simulink model "configB"  (R2022b)
settings: Solver=VariableStepAuto  StartTime=0.0  StopTime=150  RelTol=1e-3
values from neighbouring files (symbols this model uses):
  densityHydrogen = poutlet*(molarMassHydrogen/1000)/(universalGasConstant2*0.001)/OperatingTemperature    (= 0.0969930238153)    [ValveSetData.m]
  flowCoefficientValve = 1.156 * 0.32    (= 0.36992)    [ValveSetData.m]
  hysteresisValve = 0.15    [ValveSetData.m]
  molarMassHydrogen = 2.016    [ValveSetData.m]
  N2 = 6950    [ValveSetData.m]
  OperatingTemperature = T_S+27    (= 300)    [ValveSetData.m]
  responseTimeValve = 0.03    [ValveSetData.m]
  SpecificGravityHydrogen = 0.0696    [ValveSetData.m]
  universalGasConstant1 = 8.3145    [ValveSetData.m]
undefined symbols (not defined in the file or in its folder): anodeInletPathVolume
libraries: slpidlib x1
settings Model: Creator=debjani.ghosh  LastModifiedBy=debjani.ghosh
settings DataIOCC: ReturnWorkspaceOutputs=off

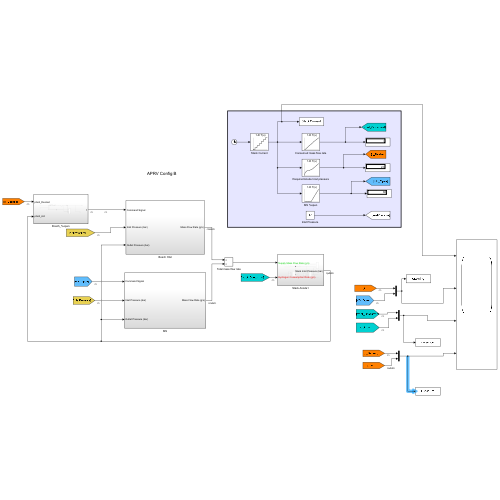
[thumbnail: Simulink's stored preview of the top-level diagram]
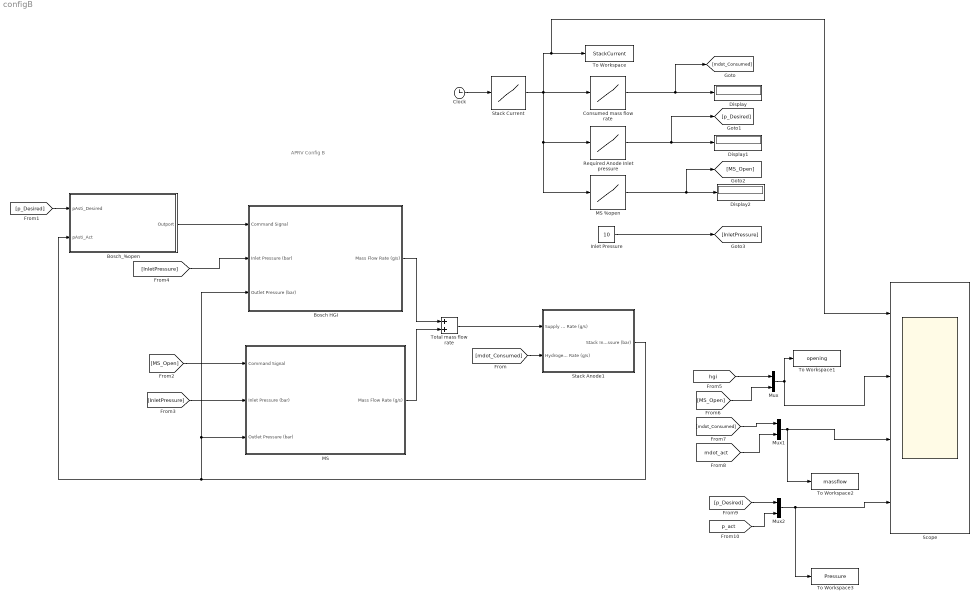
== system configB ==
  note: APRV Config B
  Bosch HGI : Subsystem
  Bosch_%open : Subsystem
  Clock : Clock
  Consumed mass flow rate : Lookup_n-D  NumberOfTableDimensions=1  BreakpointsForDimension1=[0;20;100;200;300;400;500;600]  Table=[0;0.1;0.5;1;1.5;2;2.5;3]  InternalRulePriority=Speed  RndMeth=Simplest
  Display : Display
  Display1 : Display
  Display2 : Display
  Inlet Pressure : Constant  Value=10
  MS : Subsystem
  MS %open : Lookup_n-D  NumberOfTableDimensions=1  BreakpointsForDimension1=[20,100,200,300,400,500,600]  Table=[0;0;0;0;20;40;60]  InternalRulePriority=Speed  RndMeth=Simplest
  Mux : Mux  Inputs=2
  Mux1 : Mux  Inputs=2
  Mux2 : Mux  Inputs=2
  Required Anode Inlet pressure : Lookup_n-D  NumberOfTableDimensions=1  BreakpointsForDimension1=[0;20;100;200;300;400;500;600]  Table=[1;1.4;1.6;1.7;1.8;2;2.3;2.6]  InternalRulePriority=Speed  RndMeth=Simplest
  Scope : Scope  NumInputPorts=4
  Stack Anode1 : Subsystem
  Stack Current : Lookup_n-D  NumberOfTableDimensions=1  BreakpointsForDimension1=[0;3;5.8;20;21.6;42;44;64;66;86;88;108;110;130;132;150]  Table=[0;0;20;20;100;100;200;200;300;300;400;400;500;500;600;600]  InternalRulePriority=Speed  RndMeth=Simplest
  To Workspace : ToWorkspace  VariableName=StackCurrent  SaveFormat=Structure With Time  SampleTime=-1
  To Workspace1 : ToWorkspace  VariableName=opening  SaveFormat=Structure With Time  SampleTime=-1
  To Workspace2 : ToWorkspace  VariableName=massflow  SaveFormat=Structure With Time  SampleTime=-1
  To Workspace3 : ToWorkspace  VariableName=Pressure  SaveFormat=Structure With Time  SampleTime=-1
  Total mass flow rate : Sum
  wires:
  [InletPressure] -> MS/2(Inlet Pressure (bar))
  Stack Anode1/1(Stack Inlet Pressure (bar)) -> Bosch_%open/2(pAsti_Act), Bosch HGI/3(Outlet Pressure (bar)), MS/3(Outlet Pressure (bar))
  MS/1(Mass Flow Rate (g/s)) -> Total mass flow rate/2
  Bosch_%open/1(Outport) -> Bosch HGI/1("Command Signal ")
  Bosch HGI/1(Mass Flow Rate (g/s)) -> Total mass flow rate/1
  Total mass flow rate/1 -> Stack Anode1/1(Supply Mass Flow Rate (g/s))
  Consumed mass flow rate/1 -> [mdot_Consumed], Display/1
  Required Anode Inlet pressure/1 -> [p_Desired], Display1/1
  [p_Desired] -> Bosch_%open/1(pAsti_Desired)
  [MS_Open] -> MS/1("Command Signal ")
  [mdot_Consumed] -> Stack Anode1/2(Hydrogen Consumption Rate (g/s))
  Clock/1 -> Stack Current/1
  MS %open/1 -> [MS_Open], Display2/1
  Stack Current/1 -> MS %open/1, Required Anode Inlet pressure/1, Scope/1, To Workspace/1, Consumed mass flow rate/1
  [InletPressure] -> Bosch HGI/2(Inlet Pressure (bar))
  Inlet Pressure/1 -> [InletPressure]
  Mux/1 -> To Workspace1/1, Scope/2
  [hgi] -> Mux/1
  [MS_Open] -> Mux/2
  [mdot_Consumed] -> Mux1/1
  [mdot_act] -> Mux1/2
  [p_Desired] -> Mux2/1
  Mux1/1 -> To Workspace2/1, Scope/3
  [p_act] -> Mux2/2
  Mux2/1 -> To Workspace3/1, Scope/4

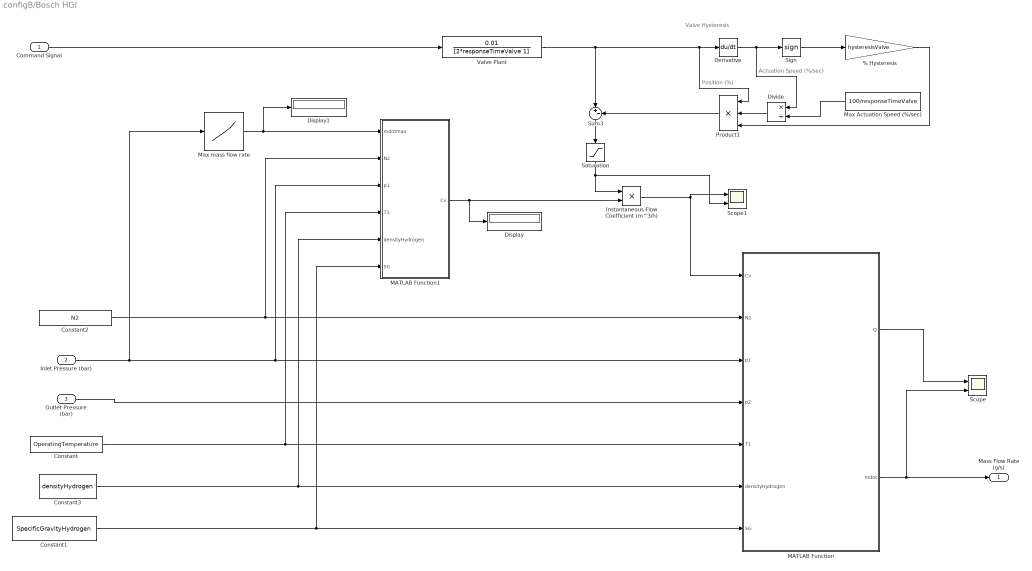
== system configB/Bosch HGI ==
  note: Actuation Speed (%/sec)
  note: Position (%)
  note: Valve Hysteresis
  "Command Signal " : Inport
  Inlet Pressure (bar) : Inport  Port=2
  Outlet Pressure (bar) : Inport  Port=3
  % Hysteresis : Gain  Gain=hysteresisValve
  Constant : Constant  Value=OperatingTemperature
  Constant1 : Constant  Value=SpecificGravityHydrogen
  Constant2 : Constant  Value=N2
  Constant3 : Constant  Value=densityHydrogen
  Derivative : Derivative
  Display : Display
  Display1 : Display
  Divide : Product  Inputs=*/
  Instantaneous Flow Coefficient (m^3/h) : Product
  MATLAB Function : MATLAB Function  TreatAsAtomicUnit=on
  MATLAB Function1 : MATLAB Function  TreatAsAtomicUnit=on
  Max Actuation Speed (%/sec) : Constant  Value=100/responseTimeValve
  Max mass flow rate : Lookup_n-D  NumberOfTableDimensions=1  BreakpointsForDimension1=[8,10,12,14,16]  Table=[1.5,1.8,2.2,2.5,2.8]  InternalRulePriority=Speed  RndMeth=Simplest
  Product1 : Product  Inputs=3
  Saturation : Saturate  UpperLimit=1  LowerLimit=0  LinearizeAsGain=off
  Scope : Scope  NumInputPorts=2
  Scope1 : Scope  NumInputPorts=2
  Sign : Signum  ZeroCross=off
  Sum3 : Sum  Inputs=|+-
  Valve Plant : TransferFcn  Numerator=0.01  Denominator=[2*responseTimeValve 1]
  Mass Flow Rate (g/s) : Outport
  wires:
  Sign/1 -> % Hysteresis/1
  Derivative/1 -> Divide/1, Sign/1
  % Hysteresis/1 -> Product1/3
  Product1/1 -> Sum3/2
  Sum3/1 -> Saturation/1
  Divide/1 -> Product1/2
  Max Actuation Speed (%/sec)/1 -> Divide/2
  Instantaneous Flow Coefficient (m^3/h)/1 -> MATLAB Function/1(Cv), Scope1/1
  Valve Plant/1 -> Sum3/1, Derivative/1, Product1/1
  "Command Signal "/1 -> Valve Plant/1
  MATLAB Function/2(mdot) -> Scope/2, Mass Flow Rate (g/s)/1
  Saturation/1 -> Scope1/2, Instantaneous Flow Coefficient (m^3/h)/1
  Constant1/1 -> MATLAB Function1/6(SG), MATLAB Function/7(SG)
  Constant/1 -> MATLAB Function/5(T1), MATLAB Function1/4(T1)
  Outlet Pressure (bar)/1 -> MATLAB Function/4(p2)
  MATLAB Function1/1(Cv) -> Display/1, Instantaneous Flow Coefficient (m^3/h)/2
  Constant2/1 -> MATLAB Function1/2(N2), MATLAB Function/2(N2)
  Inlet Pressure (bar)/1 -> Max mass flow rate/1, MATLAB Function1/3(p1), MATLAB Function/3(p1)
  Max mass flow rate/1 -> Display1/1, MATLAB Function1/1(mdotmax)
  Constant3/1 -> MATLAB Function1/5(densityHydrogen), MATLAB Function/6(densityHydrogen)
  MATLAB Function/1(Q) -> Scope/1

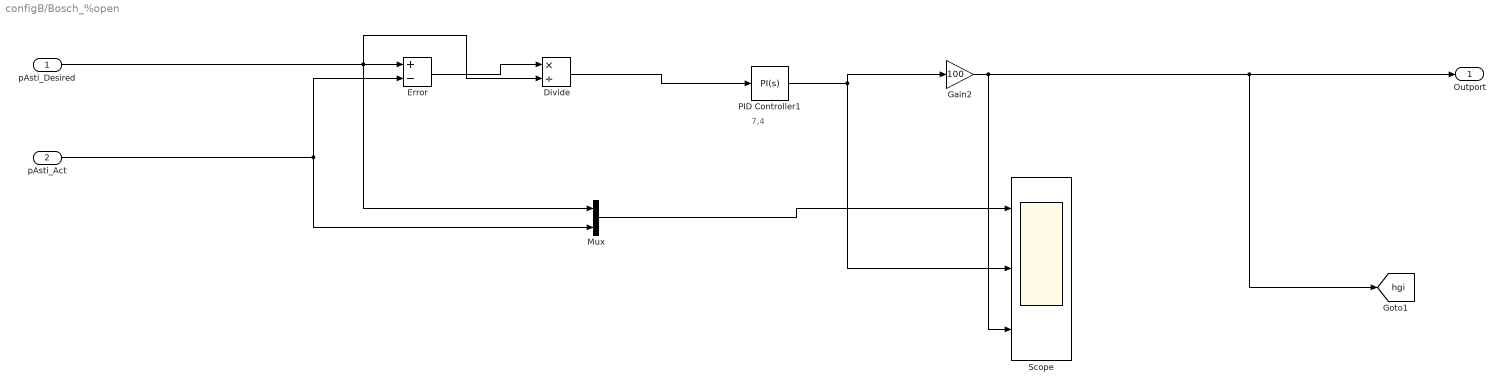
== system configB/Bosch_%open ==
  note: 7,4
  pAsti_Desired : Inport
  pAsti_Act : Inport  Port=2
  Divide : Product  Inputs=*/
  Error : Sum  Inputs=+-
  Gain2 : Gain  Gain=100
  Mux : Mux  Inputs=2
  PID Controller1 : slpidlib/PID Controller  Controller=PI  Form=Parallel  TimeDomain=Continuous-time  UseExternalTs=off  SampleTime=-1  IntegratorMethod=Forward Euler  FilterMethod=Forward Euler  ControllerParametersSource=internal  P=5  I=5  UseKiTs=on  D=0.459  N=100  UseFilter=on  TunerSelectOption=Transfer Function Based (PID Tuner App)  InitialConditionSource=internal  InitialConditionForIntegrator=0  InitialConditionForFilter=0  DifferentiatorICPrevScaledInput=0  ExternalReset=none  TrackingMode=off  Kt=1  LimitOutput=on  SatLimitsSource=internal  UpperSaturationLimit=1  LowerSaturationLimit=0  LinearizeAsGain=on  AntiWindupMode=none  Kb=1  LimitIntegrator=off  UpperIntegratorSaturationLimit=inf  LowerIntegratorSaturationLimit=-inf  POutMin=[]  POutMax=[]  IOutMin=[]  IOutMax=[]  DOutMin=[]  DOutMax=[]  NOutMin=[]  NOutMax=[]  SumOutMin=[]  SumOutMax=[]  SaturationOutMin=[]  SaturationOutMax=[]  PParamMin=[]  PParamMax=[]  IParamMin=[]  IParamMax=[]  DParamMin=[]  DParamMax=[]  NParamMin=[]  NParamMax=[]  KbParamMin=[]  KbParamMax=[]  KtParamMin=[]  KtParamMax=[]  KbOutMin=[]  KbOutMax=[]  KtOutMin=[]  KtOutMax=[]  IntegratorOutMin=[]  IntegratorOutMax=[]  FilterOutMin=[]  FilterOutMax=[]  SumI1OutMin=[]  SumI1OutMax=[]  SumI2OutMin=[]  SumI2OutMax=[]  SumI3OutMin=[]  SumI3OutMax=[]  SumI4OutMin=[]  SumI4OutMax=[]  SumDOutMin=[]  SumDOutMax=[]  DifferentiatorOutMin=[]  DifferentiatorOutMax=[]  FilterDiffOutCoefMin=[]  FilterDiffOutCoefMax=[]  ReciprocalOutMin=[]  ReciprocalOutMax=[]  SumDenOutMin=[]  SumDenOutMax=[]  SumNumOutMin=[]  SumNumOutMax=[]  DivideOutMin=[]  DivideOutMax=[]  UdiffTsProdOutMin=[]  UdiffTsProdOutMax=[]  NTsProdOutMin=[]  NTsProdOutMax=[]  UintegralTsProdOutMin=[]  UintegralTsProdOutMax=[]  UngainTsProdOutMin=[]  UngainTsProdOutMax=[]  ClampingZeroOutDataTypeStr=Inherit: Inherit via back propagation  ClampingZeroOutMin=[]  ClampingZeroOutMax=[]  FilterDenConstantOutDataTypeStr=Inherit: Inherit via back propagation  FilterDenConstantOutMin=[]  FilterDenConstantOutMax=[]  PCopyOutDataTypeStr=Inherit: Inherit via back propagation  PCopyOutMin=[]  PCopyOutMax=[]  NCopyOutDataTypeStr=Inherit: Inherit via back propagation  NCopyOutMin=[]  NCopyOutMax=[]  IntegratorContinuousStateAttributes=''  IntegratorStateMustResolveToSignalObject=off  IntegratorRTWStateStorageClass=Auto  FilterContinuousStateAttributes=''  FilterStateMustResolveToSignalObject=off  FilterRTWStateStorageClass=Auto  ParallelPVariant=InternalParameters  IdealPVariant=Disabled  IVariant=InternalParameters  DVariant=Disabled  IntegratorVariant=Continuous  SatVariant=Enabled  AWVariant=Passthrough  PCopyVariant=Disabled  TRVariant=Disabled  FdbkBlocksVariant=Forward  IdealPFdbkVariant=Disabled  SatFdbkVariant=Disabled  DerivativeFilterVariant=Disabled  NVariant=Disabled  NCopyVariant=Disabled_SignalSpec  FilterICVariant=Disabled  IntegratorICVariant=InternalICs  ExternalResetVariant=Disabled  TRSumVariant=Passthrough  SumFdbkVariant=Disabled  SumVariant=Sum_PI  TsampFilterVariant=InternalTs  TsampNgainVariant=Passthrough  TsampIntegralVariant=Passthrough  ExternalSaturationOutDataTypeStr=Inherit: Same as second input
  Scope : Scope  NumInputPorts=3
  Outport : Outport
  tag scope: hgi=global
  wires:
  Error/1 -> Divide/1
  pAsti_Act/1 -> Mux/2, Error/2
  PID Controller1/1 -> Gain2/1, Scope/2
  Mux/1 -> Scope/1
  pAsti_Desired/1 -> Mux/1, Divide/2, Error/1
  Divide/1 -> PID Controller1/1
  Gain2/1 -> Scope/3, [hgi], Outport/1

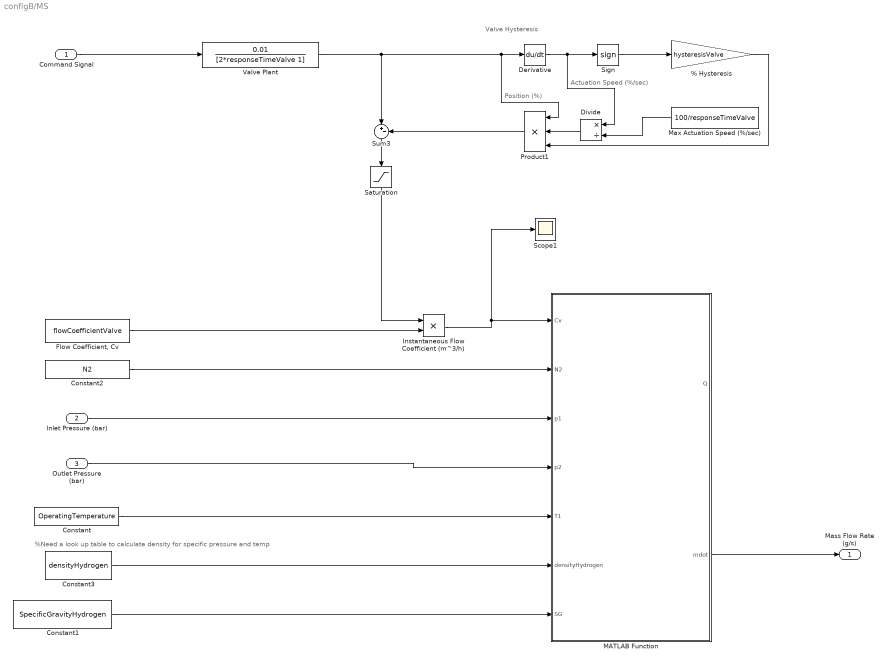
== system configB/MS ==
  note: %Need a look up table to calculate density for specific pressure and temp
  note: Actuation Speed (%/sec)
  note: Position (%)
  note: Valve Hysteresis
  "Command Signal " : Inport
  Inlet Pressure (bar) : Inport  Port=2
  Outlet Pressure (bar) : Inport  Port=3
  % Hysteresis : Gain  Gain=hysteresisValve
  Constant : Constant  Value=OperatingTemperature
  Constant1 : Constant  Value=SpecificGravityHydrogen
  Constant2 : Constant  Value=N2
  Constant3 : Constant  Value=densityHydrogen
  Derivative : Derivative
  Divide : Product  Inputs=*/
  "Flow Coefficient, Cv" : Constant  Value=flowCoefficientValve
  Instantaneous Flow Coefficient (m^3/h) : Product
  MATLAB Function : MATLAB Function  TreatAsAtomicUnit=on
  Max Actuation Speed (%/sec) : Constant  Value=100/responseTimeValve
  Product1 : Product  Inputs=3
  Saturation : Saturate  UpperLimit=1  LowerLimit=0  LinearizeAsGain=off
  Scope1 : Scope
  Sign : Signum  ZeroCross=off
  Sum3 : Sum  Inputs=|+-
  Valve Plant : TransferFcn  Numerator=[0.01]  Denominator=[2*responseTimeValve 1]
  Mass Flow Rate (g/s) : Outport
  wires:
  Sign/1 -> % Hysteresis/1
  Derivative/1 -> Divide/1, Sign/1
  "Flow Coefficient, Cv"/1 -> Instantaneous Flow Coefficient (m^3/h)/2
  % Hysteresis/1 -> Product1/3
  Product1/1 -> Sum3/2
  Sum3/1 -> Saturation/1
  Divide/1 -> Product1/2
  Max Actuation Speed (%/sec)/1 -> Divide/2
  Instantaneous Flow Coefficient (m^3/h)/1 -> Scope1/1, MATLAB Function/1(Cv)
  Valve Plant/1 -> Sum3/1, Derivative/1, Product1/1
  "Command Signal "/1 -> Valve Plant/1
  MATLAB Function/2(mdot) -> Mass Flow Rate (g/s)/1
  Saturation/1 -> Instantaneous Flow Coefficient (m^3/h)/1
  Constant1/1 -> MATLAB Function/7(SG)
  Constant/1 -> MATLAB Function/5(T1)
  Outlet Pressure (bar)/1 -> MATLAB Function/4(p2)
  Inlet Pressure (bar)/1 -> MATLAB Function/3(p1)
  Constant2/1 -> MATLAB Function/2(N2)
  Constant3/1 -> MATLAB Function/6(densityHydrogen)

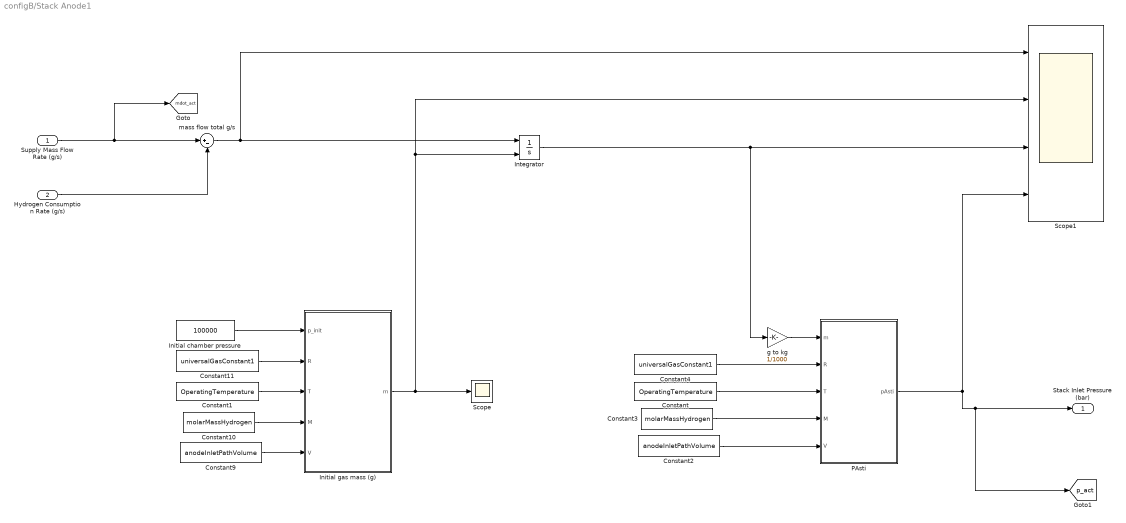
== system configB/Stack Anode1 ==
  Supply Mass Flow Rate (g/s) : Inport
  Hydrogen Consumption Rate (g/s) : Inport  Port=2
  Constant : Constant  Value=OperatingTemperature
  Constant1 : Constant  Value=OperatingTemperature
  Constant10 : Constant  Value=molarMassHydrogen
  Constant11 : Constant  Value=universalGasConstant1
  Constant2 : Constant  Value=anodeInletPathVolume
  Constant3 : Constant  Value=molarMassHydrogen
  Constant4 : Constant  Value=universalGasConstant1
  Constant9 : Constant  Value=anodeInletPathVolume
  Initial chamber pressure : Constant  Value=100000
  Initial gas mass (g) : MATLAB Function  TreatAsAtomicUnit=on
  Integrator : Integrator  InitialConditionSource=external
  PAsti : MATLAB Function  TreatAsAtomicUnit=on
  Scope : Scope
  Scope1 : Scope  NumInputPorts=4
  g to kg : Gain  Gain=1/1000
  mass flow total g/s : Sum  Inputs=|+-
  Stack Inlet Pressure (bar) : Outport
  tag scope: mdot_act=global, p_act=global
  wires:
  Initial chamber pressure/1 -> Initial gas mass (g)/1(p_init)
  Constant/1 -> PAsti/3(T)
  Constant4/1 -> PAsti/2(R)
  Constant3/1 -> PAsti/4(M)
  Constant2/1 -> PAsti/5(V)
  Constant11/1 -> Initial gas mass (g)/2(R)
  Constant1/1 -> Initial gas mass (g)/3(T)
  Constant10/1 -> Initial gas mass (g)/4(M)
  Constant9/1 -> Initial gas mass (g)/5(V)
  mass flow total g/s/1 -> Integrator/1, Scope1/1
  Hydrogen Consumption Rate (g/s)/1 -> mass flow total g/s/2
  Supply Mass Flow Rate (g/s)/1 -> [mdot_act], mass flow total g/s/1
  g to kg/1 -> PAsti/1(m)
  Initial gas mass (g)/1(m) -> Scope1/2, Integrator/2, Scope/1
  Integrator/1 -> g to kg/1, Scope1/3
  PAsti/1(pAsti) -> Scope1/4, [p_act], Stack Inlet Pressure (bar)/1

== matlab function configB/Bosch HGI/MATLAB Function1 ==
  data: mdotmax input; Cv output; N2 input; p1 input; T1 input; densityHydrogen input; SG input
function Cv = fcn(mdotmax,N2, p1,T1,densityHydrogen, SG)

Q = mdotmax /(0.06 * densityHydrogen* 1000/3600);

Cv = Q / (0.471*N2*p1*sqrt(1/(SG*T1)));

== matlab function configB/Bosch HGI/MATLAB Function ==
  data: Q output; Cv input; N2 input; p1 input; p2 input; T1 input; densityHydrogen input; mdot output; SG input
function [Q,mdot]   = fcn(Cv, N2, p1,p2, T1,densityHydrogen, SG)
%Calculation of mass flow based on Swagelok 
% Valve Sizing Technical Bulletin


%Calculate pressure difference between inlet and outlet

dp = p1-p2;

if p2 > p1/2

     % low pressure drop - subsonic flow

    Q = N2*Cv*p1*(1-(2*dp)/(3*p1))*sqrt(dp/(p1*SG*T1)); % standard volumetric flow rate in lpm 

else
   
    % high pressure drop - sonic flow (independent of downstream pressure)

    Q =  0.471*N2*Cv*p1*sqrt(1/(SG*T1)); % standard volumetric flow rate in lpm  

end

   %Comment: densityHydrogen must be a value dependent on operating T and p

    mdot = 0.06* Q * densityHydrogen* 1000/3600;  %g/s

    %Volumetric flow rate in lpm @ operating T and p
    % T1=T2

   % Vdot = Q * 1.01 * T1 /( p2 * 273);  % lpm

== matlab function configB/MS/MATLAB Function ==
  data: Q output; Cv input; N2 input; p1 input; p2 input; T1 input; densityHydrogen input; mdot output; SG input
function [Q,mdot]   = fcn(Cv, N2, p1,p2, T1,densityHydrogen, SG)
%Calculation of mass flow based on Swagelok 
% Valve Sizing Technical Bulletin


%Calculate pressure difference between inlet and outlet

dp = p1-p2;

if p2 > p1/2

     % low pressure drop - subsonic flow

    Q = N2*Cv*p1*(1-(2*dp)/(3*p1))*sqrt(dp/(p1*SG*T1)); % standard volumetric flow rate in lpm 

else
   
    % high pressure drop - sonic flow (independent of downstream pressure)

    Q =  0.471*N2*Cv*p1*sqrt(1/(SG*T1)); % standard volumetric flow rate in lpm  

end

   %Comment: densityHydrogen must be a value dependent on operating T and p

    mdot = 0.06* Q * densityHydrogen* 1000/3600;  %g/s

    %Volumetric flow rate in lpm @ operating T and p
    % T1=T2

   % Vdot = Q * 1.01 * T1 /( p2 * 273);  % lpm

== matlab function configB/Stack Anode1/Initial gas mass (g) ==
  data: p_init input; m output; R input; T input; M input; V input
function m = fcn(p_init,R,T,M,V)

%from Ideal Gas Law

m = 1000*((p_init * M * V) / (R * T));  %mass in g

== matlab function configB/Stack Anode1/PAsti ==
  data: m input; pAsti output; R input; T input; M input; V input
function pAsti = fcn(m,R,T,M,V)

%from Ideal Gas Law

p = (m * R * T) / (M * V);  %Pressure in Pa

pAsti =p * 1e-5;  % Pressure in bar
